simulink model "g_z_cl_old"  (Simulink 5.0)
settings: Solver=ode45  StartTime=t0  StopTime=tf  RelTol=1e-3
values from neighbouring files (symbols this model uses):
  A = den    [d2filt.m]
  B = num    [d2filt.m]
undefined symbols (not defined in the file or in its folder): C, D, D1, N1, N_var, R, S, st, T, Ts, zk
settings Model: Creator=kannan  LastModifiedBy=kannan  ExtModeAutoUpdateStatusClock=off

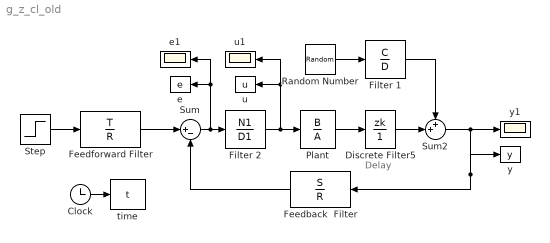
== system g_z_cl_old ==
  note: Delay
  " Filter 2" : DiscreteFilter  Numerator=N1  Denominator=D1  SampleTime=Ts
  Clock : Clock
      settings: Decimation=10
  Discrete Filter5 : DiscreteFilter  Numerator=zk  Denominator=1  SampleTime=Ts
  Feedback  Filter : DiscreteFilter  Orientation=left  Numerator=S  Denominator=R  SampleTime=Ts
  Feedforward Filter : DiscreteFilter  Numerator=T  Denominator=R  SampleTime=Ts
  Filter 1 : DiscreteFilter  Numerator=C  Denominator=D  SampleTime=Ts
  Plant : DiscreteFilter  Numerator=B  Denominator=A  SampleTime=Ts
  Random Number : RandomNumber  Variance=N_var  SampleTime=Ts
  Step : Step  Time=0  After=st  SampleTime=Ts
  Sum : Sum  Inputs=|+-  SaturateOnIntegerOverflow=on
  Sum2 : Sum  Inputs=++|  SaturateOnIntegerOverflow=on
  e : ToWorkspace  VariableName=e  SampleTime=Ts  SaveFormat=Array
  e1 : Scope
      settings: YMin=-6e+164  YMax=1.02293e+149  SaveName=ScopeData2
  time : ToWorkspace  VariableName=t  SampleTime=Ts  SaveFormat=Array
  u : ToWorkspace  VariableName=u  SampleTime=Ts  SaveFormat=Array
  u1 : Scope
      settings: YMin=-6e+164  YMax=1.02293e+149
  y : ToWorkspace  VariableName=y  SampleTime=Ts  SaveFormat=Array
  y1 : Scope
      settings: YMin=-6e+164  YMax=1.02293e+149
  wires:
  Step/1 -> Feedforward Filter/1
  Feedforward Filter/1 -> Sum/1
  Feedback  Filter/1 -> Sum/2
  Clock/1 -> time/1
  Plant/1 -> Discrete Filter5/1
  Discrete Filter5/1 -> Sum2/2
  Filter 1/1 -> Sum2/1
  Random Number/1 -> Filter 1/1
  Sum2/1 -> y1/1, Feedback  Filter/1, y/1
  Sum/1 -> " Filter 2"/1, e/1, e1/1
  " Filter 2"/1 -> Plant/1, u1/1, u/1
